simulink model "SSBSC generation"  (R2022b)
settings: Solver=VariableStepAuto  StartTime=0.0  StopTime=0.001  RelTol=1e-3
libraries: dsparch4 x1
settings Model: Creator=mluser  LastModifiedBy=mluser

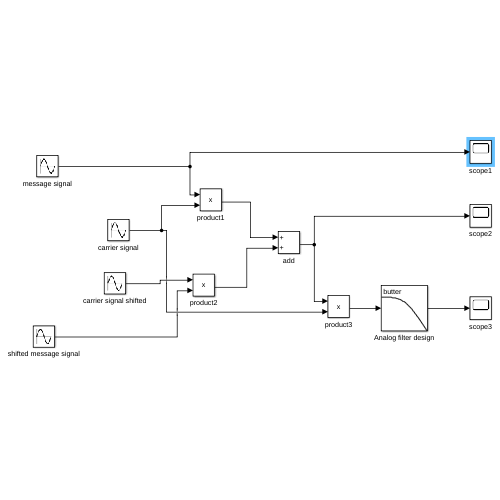
[thumbnail: Simulink's stored preview of the top-level diagram]
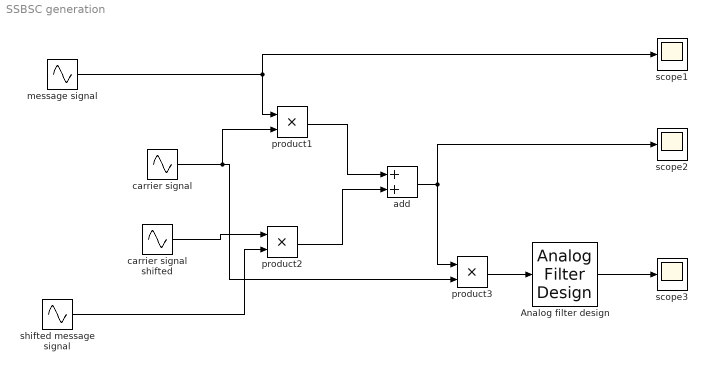
== system SSBSC generation ==
  "Analog filter design " : dsparch4/Analog Filter Design  method=Butterworth  filttype=Lowpass  N=1  Wlo=2*pi*2000  Whi=80  Rp=2  Rs=40
  add : Sum
  carrier signal : Sin  Frequency=2*pi*100000  Phase=-(pi/2)  SampleTime=0
  carrier signal shifted : Sin  Frequency=2*pi*100000  SampleTime=0
  message signal : Sin  Frequency=2*pi*2000  SampleTime=0
  product1 : Product
  product2 : Product
  product3 : Product
  scope1 : Scope
  scope2 : Scope
  "scope3 " : Scope
  shifted message signal : Sin  Frequency=2*pi*2000  Phase=-(pi/2)  SampleTime=0
  wires:
  carrier signal/1 -> product3/2, product1/2
  carrier signal shifted/1 -> product2/1
  shifted message signal/1 -> product2/2
  product1/1 -> add/1
  product2/1 -> add/2
  add/1 -> scope2/1, product3/1
  message signal/1 -> scope1/1, product1/1
  product3/1 -> "Analog filter design "/1
  "Analog filter design "/1 -> "scope3 "/1
